simulink model "dekf_estimate"  (R2021a)
settings: Solver=VariableStepAuto  StartTime=0.0  StopTime=time_est  RelTol=1e-3
values from neighbouring files (symbols this model uses):
  Delta = block.DialogPrm(1).Data    [battery_dual_ekf_2.m]    (also in init_dekf_2.m = 0.008)
settings Model: Creator=saleh  LastModifiedBy=saleh

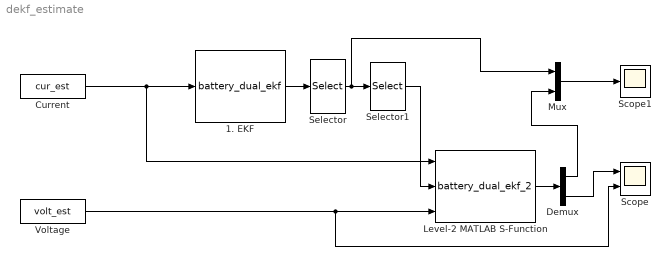
== system dekf_estimate ==
  1. EKF : M-S-Function  FunctionName=battery_dual_ekf  Parameters=Delta, x_0, P_0, a, Z_k, W_k, Qe, Cg
  Current : FromWorkspace  VariableName=cur_est  SampleTime=Delta
  Demux : Demux  Outputs=2
  Level-2 MATLAB S-Function : M-S-Function  FunctionName=battery_dual_ekf_2  Parameters=Delta, x_b_0, P_b_0, Z_b_k, W_b_k, Cg
  Mux : Mux  Inputs=2
  Scope : Scope  NumInputPorts=2
  Scope1 : Scope
  Selector : Selector  InputPortWidth=8  IndexOptions=Index vector (dialog)  Indices=[1:6]  OutputSizes=1
  Selector1 : Selector  InputPortWidth=6  IndexOptions=Index vector (dialog)  Indices=[6]  OutputSizes=1
  Voltage : FromWorkspace  VariableName=volt_est  SampleTime=Delta
  wires:
  Current/1 -> Level-2 MATLAB S-Function/1, 1. EKF/1
  Voltage/1 -> Scope/2, Level-2 MATLAB S-Function/3
  1. EKF/1 -> Selector/1
  Level-2 MATLAB S-Function/1 -> Demux/1
  Demux/2 -> Scope/1
  Selector/1 -> Mux/1, Selector1/1
  Selector1/1 -> Level-2 MATLAB S-Function/2
  Demux/1 -> Mux/2
  Mux/1 -> Scope1/1
